simulink model "stabilization2311"  (R2024a)
settings: Solver=VariableStepAuto  StartTime=0.0  StopTime=10  RelTol=1e-3
settings Model: Creator=pupkinzalupkin  LastModifiedBy=pupkinzalupkin

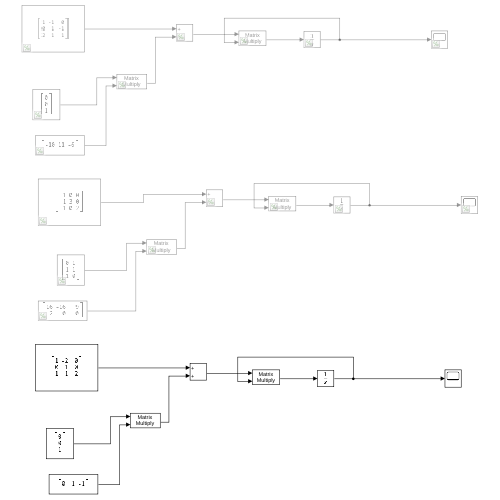
[thumbnail: Simulink's stored preview of the top-level diagram]
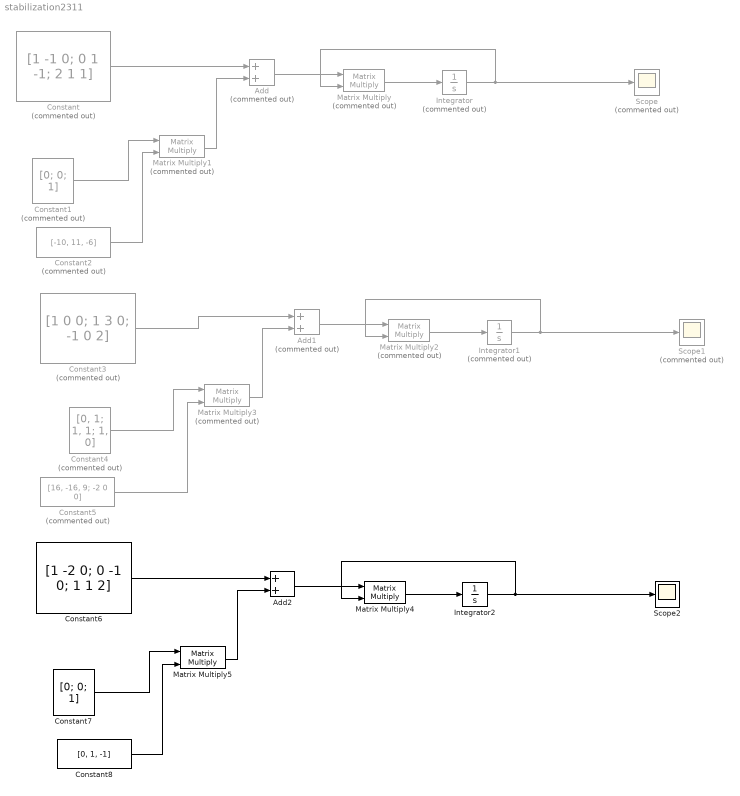
== system stabilization2311 ==
  Add : Sum  Commented=on
  Add1 : Sum  Commented=on
  Add2 : Sum
  Constant : Constant  Commented=on  Value=[1 -1 0; 0 1 -1; 2 1 1]
  Constant1 : Constant  Commented=on  Value=[0; 0; 1]  VectorParams1D=off
  Constant2 : Constant  Commented=on  Value=[-10, 11, -6]  VectorParams1D=off
  Constant3 : Constant  Commented=on  Value=[1 0 0; 1 3 0; -1 0 2]
  Constant4 : Constant  Commented=on  Value=[0, 1; 1, 1; 1, 0]  VectorParams1D=off
  Constant5 : Constant  Commented=on  Value="[16,  -16, 9; -2 0 0]"  VectorParams1D=off
  Constant6 : Constant  Value=[1 -2 0; 0 -1 0; 1 1 2]
  Constant7 : Constant  Value=[0; 0; 1]  VectorParams1D=off
  Constant8 : Constant  Value=[0, 1, -1]  VectorParams1D=off
  Integrator : Integrator  Commented=on  InitialCondition=[0; 0; -1]
  Integrator1 : Integrator  Commented=on  InitialCondition=[0; 0; -1]
  Integrator2 : Integrator  InitialCondition=[0; 0; -1]
  Matrix Multiply{,1..3} (4 alike) : Product  Commented=on  Multiplication=Matrix(*)
  Matrix Multiply4 : Product  Multiplication=Matrix(*)
  Matrix Multiply5 : Product  Multiplication=Matrix(*)
  Scope : Scope  Commented=on
  Scope1 : Scope  Commented=on
  Scope2 : Scope
  wires:
  Matrix Multiply/1 -> Integrator/1
  Integrator/1 -> Matrix Multiply/2, Scope/1
  Constant/1 -> Add/1
  Add/1 -> Matrix Multiply/1
  Constant1/1 -> Matrix Multiply1/1
  Constant2/1 -> Matrix Multiply1/2
  Matrix Multiply1/1 -> Add/2
  Matrix Multiply3/1 -> Add1/2
  Constant5/1 -> Matrix Multiply3/2
  Matrix Multiply2/1 -> Integrator1/1
  Add1/1 -> Matrix Multiply2/1
  Integrator1/1 -> Matrix Multiply2/2, Scope1/1
  Constant4/1 -> Matrix Multiply3/1
  Constant3/1 -> Add1/1
  Matrix Multiply5/1 -> Add2/2
  Constant8/1 -> Matrix Multiply5/2
  Matrix Multiply4/1 -> Integrator2/1
  Add2/1 -> Matrix Multiply4/1
  Integrator2/1 -> Matrix Multiply4/2, Scope2/1
  Constant7/1 -> Matrix Multiply5/1
  Constant6/1 -> Add2/1
